simulink model "heat_exchange_step_general"  (R2018b)
settings: Solver=ode23s  StartTime=0.0  StopTime=4  RelTol=1e-3
values from neighbouring files (symbols this model uses):
  f = 1    [temp_control_cstr.m]
  f0 = 2    [temp_control_cstr.m]
  k1 = 1    [temp_control_cstr.m]
  K1 = yfinal/2    (= 1.055)    [temp_control_cstr.m]
  k2 = 1    [temp_control_cstr.m]
  k3 = 4    [temp_control_cstr.m]
  k4 = 6    [temp_control_cstr.m]
  T0 = f*k1/(f*k1+k2) * Ti + k2/(f*k1+k2)*Th0    (= 36.4545454545)    [temp_control_cstr.m]
  T1 = params(2)    [temp_control_cstr.m]
  tau1 = params(1)    [temp_control_cstr.m]
  Th0 = f0*k3/den_Th*Ts +      k4*f*k1/(f*k1+k2) / den_Th * Ti    (= 49.9090909091)    [temp_control_cstr.m]
  Ti = 23    [temp_control_cstr.m]
  Ts = 60    [temp_control_cstr.m]
settings Model: Creator=kjartan  LastModifiedBy=kjartan

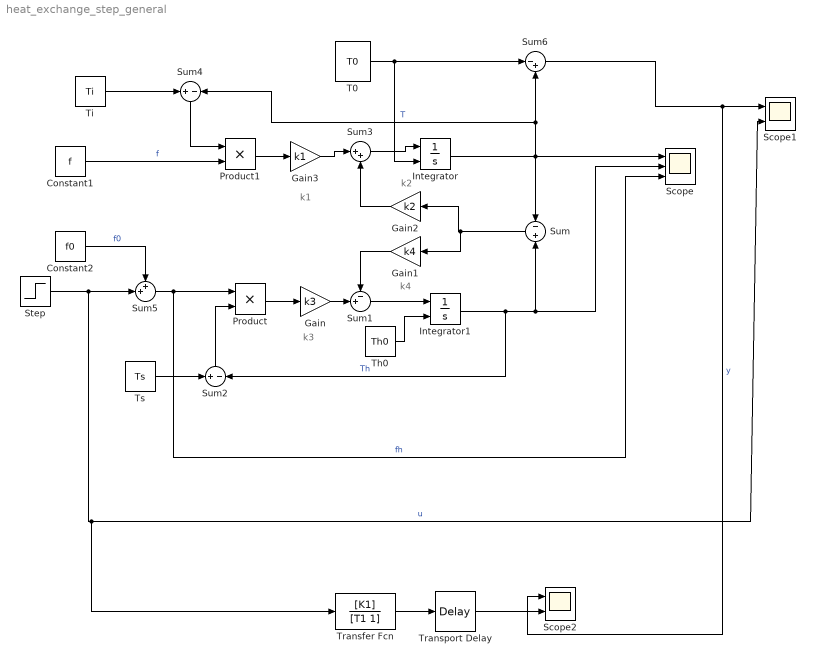
== system heat_exchange_step_general ==
  note: k3
  note: k4
  note: k2
  note: k1
  Constant1 : Constant  Value=f
  Constant2 : Constant  Value=f0
  Gain : Gain  Gain=k3
  Gain1 : Gain  Gain=k4
  Gain2 : Gain  Gain=k2
  Gain3 : Gain  Gain=k1
  Integrator : Integrator  InitialConditionSource=external  InitialCondition=1.4
  Integrator1 : Integrator  InitialConditionSource=external  InitialCondition=1.8
  Product : Product
  Product1 : Product
  Scope : Scope  NumInputPorts=3
  Scope1 : Scope  NumInputPorts=2
  Scope2 : Scope  NumInputPorts=2
  Step : Step  After=2  SampleTime=0
  Sum : Sum  Inputs=-|+
  Sum1 : Sum  Inputs=-+|
  Sum2 : Sum  Inputs=+|-
  Sum3 : Sum  Inputs=|++
  Sum4 : Sum  Inputs=+|-
  Sum5 : Sum  Inputs=++|
  Sum6 : Sum  Inputs=|-+
  T0 : Constant  Value=T0
  Th0 : Constant  Value=Th0
  Ti : Constant  Value=Ti
  Transfer Fcn : TransferFcn  Numerator=[K1]  Denominator=[T1 1]
  Transport Delay : TransportDelay  DelayTime=tau1
  Ts : Constant  Value=Ts
  wires:
  Integrator1/1 -> Scope/2, Sum/2, Sum2/2  "Th"
  Product/1 -> Gain/1
  Sum1/1 -> Integrator1/1
  Gain/1 -> Sum1/2
  Sum/1 -> Gain1/1, Gain2/1
  Gain1/1 -> Sum1/1
  Ts/1 -> Sum2/1
  Sum2/1 -> Product/2
  Sum3/1 -> Integrator/1
  Gain2/1 -> Sum3/2
  Ti/1 -> Sum4/1
  Sum4/1 -> Product1/1
  Gain3/1 -> Sum3/1
  Step/1 -> Sum5/2, Transfer Fcn/1, Scope1/2  "u"
  Constant2/1 -> Sum5/1  "f0"
  Sum5/1 -> Scope/3, Product/1  "fh"
  T0/1 -> Integrator/2, Sum6/1
  Th0/1 -> Integrator1/2
  Integrator/1 -> Sum/1, Scope/1, Sum4/2, Sum6/2  "T"
  Sum6/1 -> Scope2/1, Scope1/1  "y"
  Product1/1 -> Gain3/1
  Constant1/1 -> Product1/2  "f"
  Transfer Fcn/1 -> Transport Delay/1
  Transport Delay/1 -> Scope2/2
